simulink model "MSM_strain_wave_actuator"  (R2024b)
settings: Solver=ode23t  StartTime=0.0  StopTime=SIMULATION_TIME  FixedStep=MAX_TIME_STEP  MaxStep=MAX_TIME_STEP  RelTol=1e-3  AbsTol=1e-3  EnableMultiTasking=on
PreLoadFcn:
  | linear_mechanism = Simulink.Variant('motion_type == "linear"');
  | rotary_mechanism = Simulink.Variant('motion_type == "rotary"');
values from neighbouring files (symbols this model uses):
  action = round(out.position_data.Data(:,5))    [msm_tooth_training_run.m]
  contact_ratio = tooth_plates_cnt / (2 * (t_a / t_b + 1))    (= 2)    [MSM_mechanism_simulation_properties.m]
  contraction_initial = -msm_length * e_initial    (= -0.001)    [MSM_mechanism_simulation_properties.m]
  controller_type_vec = zeros(tooth_plates_cnt, 1)    [MSM_mechanism_simulation_properties.m]
  controller_velocity_setpoint = velocity_iter    [controller_mass_comparison_runs.m]
  disk_diameter = disk_teeth_count * tooth_pitch / pi    [MSM_mechanism_simulation_properties.m]    (also in msm_sim_runs_for_pid.m = evalin('base','disk_diameter'); save_sim_result.m = evalin('base','disk_diameter'))
  disk_height = 2.5e-4    (= 0.00025)    [MSM_mechanism_simulation_properties.m]    (also in get_tooth_properties.m)
  feedback_threshold = 1.025    [MSM_mechanism_simulation_properties.m]    (also in get_tooth_properties.m; msm_sim_runs_for_pid.m = evalin('base','feedback_threshold'))
  force_control_coeff = 1.0    (= 1)    [MSM_mechanism_simulation_properties.m]
  HALT_VELOCITY = 0.2    [MSM_mechanism_simulation_properties.m]    (also in get_tooth_properties.m)
  in_pair_angle_tooth_plates_pitch = 2*pi * (-2*tooth_pitch + in_pair_tooth_plates_pitch) / (pi*disk_diameter)    (= 0.412285714286)    [MSM_mechanism_simulation_properties.m]    (also in get_tooth_properties.m = 2*pi * (-2*tooth_pitch + in_pair_tooth_plates_pitch) / (pi*t)
  MAX_OVERLOAD_VELOCITY = 100    [MSM_mechanism_simulation_properties.m]    (also in get_tooth_properties.m)
  MAX_POSITION = rack_initial_position + max_teeth_passed * tooth_plates_cnt * angle_single_tooth_step    [MSM_mechanism_simulation_properties.m]    (also in get_tooth_properties.m)
  MAX_TIME_STEP = 5e-6    (= 5e-06)    [MSM_mechanism_simulation_properties.m]
  min_tooth_motion_range = -msm_length * allowed_elongation    (= -0.001)    [MSM_mechanism_simulation_properties.m]
  motion_type_number = NaN    [MSM_mechanism_simulation_properties.m]
  next_vec_fraction = -0.05    [MSM_mechanism_simulation_properties.m]    (also in msm_sim_runs_for_pid.m = evalin('base','next_vec_fraction'))
  obs_matrix = zeros(tooth_plates_cnt, obs_matrix_size)    [MSM_mechanism_simulation_properties.m]
  one_side_absolute_offset = one_side_elongation_capacity * msm_length    (= 0.0001)    [MSM_mechanism_simulation_properties.m]
  rack_coulumb_friction = 0.05    [MSM_mechanism_simulation_properties.m]
  rack_initial_position = rack_initial_position + 4*angle_single_tooth_step    (= 0.0554357142857)    [MSM_mechanism_simulation_properties.m]    (also in get_tooth_properties.m = rack_initial_position + 4*angle_single_tooth_step)
  rack_mass = 4e-3    (= 0.004)    [MSM_mechanism_simulation_properties.m]
  rotational_rack_coulumb_friction = rack_coulumb_friction * disk_diameter    (= 0.00175)    [MSM_mechanism_simulation_properties.m]
  SIMULATION_TIME = 0.06    [MSM_mechanism_simulation_properties.m]    (also in msm_actuation_time_sensetivity.m = 0.04; msm_sim_runs_for_pid.m = evalin('base','SIMULATION_TIME'); msm_simulation_run.m = 0.08; msm_tooth_training_run.m = 0.04)
  swing_block_tooth_plates_pitch = 2 * tooth_pitch * 22 + tooth_pitch / tooth_plates_cnt    (= 0.0172575)    [MSM_mechanism_simulation_properties.m]    (also in get_tooth_properties.m = 2 * tooth_pitch * 22 + tooth_pitch / tooth_plates_cnt)
  tooth_disk_mass = 5e-3    (= 0.005)    [MSM_mechanism_simulation_properties.m]
  tooth_pitch = tooth_pitch * tooth_size_modifier    (= 0.00039)    [MSM_mechanism_simulation_properties.m]    (also in get_tooth_properties.m = 0.00024661; msm_sim_runs_for_pid.m = evalin('base','tooth_pitch'); save_sim_result.m = evalin('base','tooth_pitch'))
  tooth_plates_cnt = 4    [MSM_mechanism_simulation_properties.m]    (also in MSM_simulation_data_processing.m = sim_data.tooth_plates_cnt; msm_actuation_time_sensetivity.m = plates_cnt_iter; msm_sim_runs_for_pid.m = evalin('base','tooth_plates_cnt'); msm_simulation_run.m = plates_cnt_iter)
  tooth_plates_pitch = tooth_pitch * 12 + tooth_pitch / tooth_plates_cnt    (= 0.0047775)    [MSM_mechanism_simulation_properties.m]    (also in get_tooth_properties.m = tooth_pitch * 12 + tooth_pitch / tooth_plates_cnt)
  useful_load = -2    [MSM_mechanism_simulation_properties.m]    (also in controller_mass_comparison_runs.m)
  useful_mass = 0.0001    [MSM_mechanism_simulation_properties.m]    (also in controller_mass_comparison_runs.m = 0.025)
  VALIDATION_START_TIME = 0.25*SIMULATION_TIME    (= 0.015)    [MSM_mechanism_simulation_properties.m]
  Z = griddata(x,y,z,X,Y)    [MSM_simulation_data_processing.m]
undefined symbols (not defined in the file or in its folder): controller_amplitude_setpoint, controller_desired_profile_type, controller_frequency_setpoint, controller_loop_type, enable_neighbours_obs, enable_vel_setpoint, external_control_value, has_external_controller, initial_spike_force, random_delay_probablity, random_switch_probability, sim_state_code, simulation_pause_time, X, Y
libraries: sm_lib x141, MSM_element x72, Flat_tooth_plate x36, Rotary_tooth_plate x36, Swing_mechanism x18, nesl_utility x16, simulink x10, fl_lib x9, rllib x7, spsMeanLib x2, slctrl_autotuning x2, slpidlib x1
(part 4 of 7)

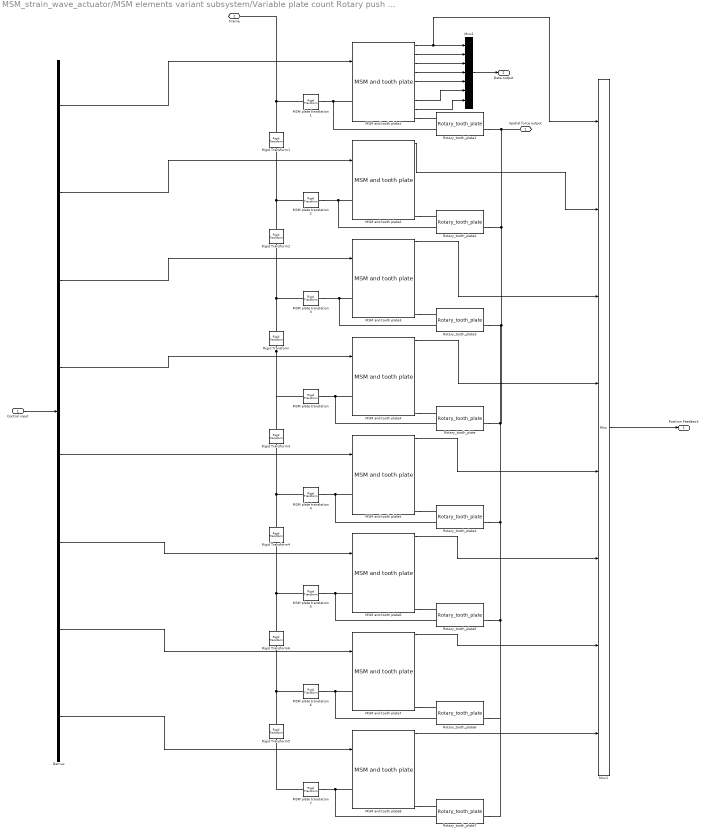
== system MSM_strain_wave_actuator/MSM elements variant subsystem/Variable plate count Rotary push spring plates/Rotary push spring 8 plates ==
  Control input : Inport
  Demux : Demux  Outputs=8
  MSM and tooth plate{1..8} (8 alike) : MSM_element/MSM and tooth plate  PositionTargetValue=contraction_initial
  MSM plate translation{,1..7} (8 alike) : sm_lib/Frames and Transforms/Rigid Transform  TranslationMethod=StandardAxis  TranslationStandardOffset=disk_diameter / 2  TranslationStandardOffsetUnits=m  TranslationStandardAxis=+Y  TranslationCartesianOffset=[0 0 0]  TranslationCartesianOffsetUnits=m  TranslationROffset=0  TranslationROffsetUnits=m  TranslationZOffset=0  TranslationZOffsetUnits=m  TranslationThetaOffset=0  TranslationThetaOffsetUnits=deg  RotationMethod=StandardAxis  RotationAngleUnits=deg  RotationStandardAxis=-X  RotationAngle=90  RotationArbitraryAxis=[0 0 1]  FollAlignAxisA=+X  BaseAlignAxisA=+Y  FollAlignAxisB=+Y  BaseAlignAxisB=+Z  RotationSequenceAxes=FollowerAxes  RotationSequence=XYX  RotationSequenceAngles=[0 0 0]  RotationSequenceAnglesUnits=deg  RotationMatrix=[1 0 0; 0 1 0; 0 0 1]  Quaternion=[1 0 0 0]
  Mux1 : Mux  Inputs=8
  Mux2 : Mux  Inputs=7
  Rigid Transform{,1..6} (7 alike) : sm_lib/Frames and Transforms/Rigid Transform  TranslationMethod=None  TranslationStandardOffset=0  TranslationStandardOffsetUnits=m  TranslationStandardAxis=+Z  TranslationCartesianOffset=[0 0 0]  TranslationCartesianOffsetUnits=m  TranslationROffset=0  TranslationROffsetUnits=m  TranslationZOffset=0  TranslationZOffsetUnits=m  TranslationThetaOffset=0  TranslationThetaOffsetUnits=deg  RotationMethod=StandardAxis  RotationAngleUnits=rad  RotationStandardAxis=+Z  RotationAngle=angle_tooth_plates_pitch  RotationArbitraryAxis=[0 0 1]  FollAlignAxisA=+X  BaseAlignAxisA=+Y  FollAlignAxisB=+Y  BaseAlignAxisB=+Z  RotationSequenceAxes=FollowerAxes  RotationSequence=XYX  RotationSequenceAngles=[0 0 0]  RotationSequenceAnglesUnits=deg  RotationMatrix=[1 0 0; 0 1 0; 0 0 1]  Quaternion=[1 0 0 0]
  Rotary_tooth_plate{,1..7} (8 alike) : Rotary_tooth_plate/Rotary_tooth_plate  SystemSampleTime=-1  VariantActivationTime=update diagram  AllowFlexibleInterface=on  Latency=0  AutoFrameSizeCalculation=off
  Spatial force output : PMIOPort  Side=Right
  Frame : PMIOPort  Port=2  Side=Left
  Position Feedback : Outport
  Data output : Outport  Port=2
  wires:
  Demux/4 -> MSM and tooth plate4/1
  MSM and tooth plate2/1 -> Mux1/2
  Control input/1 -> Demux/1
  Mux1/1 -> Position Feedback/1
  Demux/3 -> MSM and tooth plate3/1
  MSM and tooth plate4/1 -> Mux1/4
  Demux/1 -> MSM and tooth plate1/1
  Demux/2 -> MSM and tooth plate2/1
  MSM and tooth plate3/1 -> Mux1/3
  MSM and tooth plate1/1 -> Mux2/1, Mux1/1
  Demux/5 -> MSM and tooth plate5/1
  Demux/6 -> MSM and tooth plate6/1
  MSM and tooth plate5/1 -> Mux1/5
  MSM and tooth plate6/1 -> Mux1/6
  Demux/7 -> MSM and tooth plate7/1
  Demux/8 -> MSM and tooth plate8/1
  MSM and tooth plate7/1 -> Mux1/7
  MSM and tooth plate8/1 -> Mux1/8
  Mux2/1 -> Data output/1
  MSM and tooth plate1/2 -> Mux2/2
  MSM and tooth plate1/3 -> Mux2/3
  MSM and tooth plate1/4 -> Mux2/4
  MSM and tooth plate1/5 -> Mux2/5
  MSM and tooth plate1/7 -> Mux2/6
  MSM and tooth plate1/8 -> Mux2/7
  connections:
  MSM plate translation/RConn1 -- Rotary_tooth_plate/LConn2 -- MSM and tooth plate4/LConn1
  MSM plate translation3/LConn1 -- Rigid Transform/LConn1 -- Rigid Transform2/RConn1
  MSM plate translation1/LConn1 -- Frame/RConn1 -- Rigid Transform1/LConn1
  Rotary_tooth_plate1/RConn1 -- Spatial force output/RConn1 -- Rotary_tooth_plate2/RConn1 -- Rotary_tooth_plate3/RConn1 -- Rotary_tooth_plate/RConn1 -- Rotary_tooth_plate7/RConn1 -- Rotary_tooth_plate6/RConn1 -- Rotary_tooth_plate5/RConn1 -- Rotary_tooth_plate4/RConn1
  MSM and tooth plate4/RConn1 -- Rotary_tooth_plate/LConn1
  MSM and tooth plate1/RConn1 -- Rotary_tooth_plate1/LConn1
  Rotary_tooth_plate1/LConn2 -- MSM plate translation1/RConn1 -- MSM and tooth plate1/LConn1
  MSM plate translation2/LConn1 -- Rigid Transform2/LConn1 -- Rigid Transform1/RConn1
  MSM and tooth plate2/RConn1 -- Rotary_tooth_plate2/LConn1
  Rigid Transform/RConn1 -- MSM plate translation/LConn1 -- Rigid Transform3/LConn1
  MSM and tooth plate3/RConn1 -- Rotary_tooth_plate3/LConn1
  MSM plate translation3/RConn1 -- Rotary_tooth_plate3/LConn2 -- MSM and tooth plate3/LConn1
  MSM plate translation2/RConn1 -- Rotary_tooth_plate2/LConn2 -- MSM and tooth plate2/LConn1
  Rotary_tooth_plate4/LConn2 -- MSM and tooth plate5/LConn1 -- MSM plate translation4/RConn1
  Rigid Transform4/LConn1 -- MSM plate translation4/LConn1 -- Rigid Transform3/RConn1
  MSM and tooth plate5/RConn1 -- Rotary_tooth_plate4/LConn1
  Rotary_tooth_plate5/LConn2 -- MSM and tooth plate6/LConn1 -- MSM plate translation5/RConn1
  MSM plate translation5/LConn1 -- Rigid Transform6/LConn1 -- Rigid Transform4/RConn1
  MSM and tooth plate6/RConn1 -- Rotary_tooth_plate5/LConn1
  MSM plate translation6/LConn1 -- Rigid Transform5/LConn1 -- Rigid Transform6/RConn1
  MSM plate translation7/RConn1 -- Rotary_tooth_plate7/LConn2 -- MSM and tooth plate8/LConn1
  MSM plate translation6/RConn1 -- Rotary_tooth_plate6/LConn2 -- MSM and tooth plate7/LConn1
  MSM plate translation7/LConn1 -- Rigid Transform5/RConn1
  MSM and tooth plate8/RConn1 -- Rotary_tooth_plate7/LConn1
  MSM and tooth plate7/RConn1 -- Rotary_tooth_plate6/LConn1

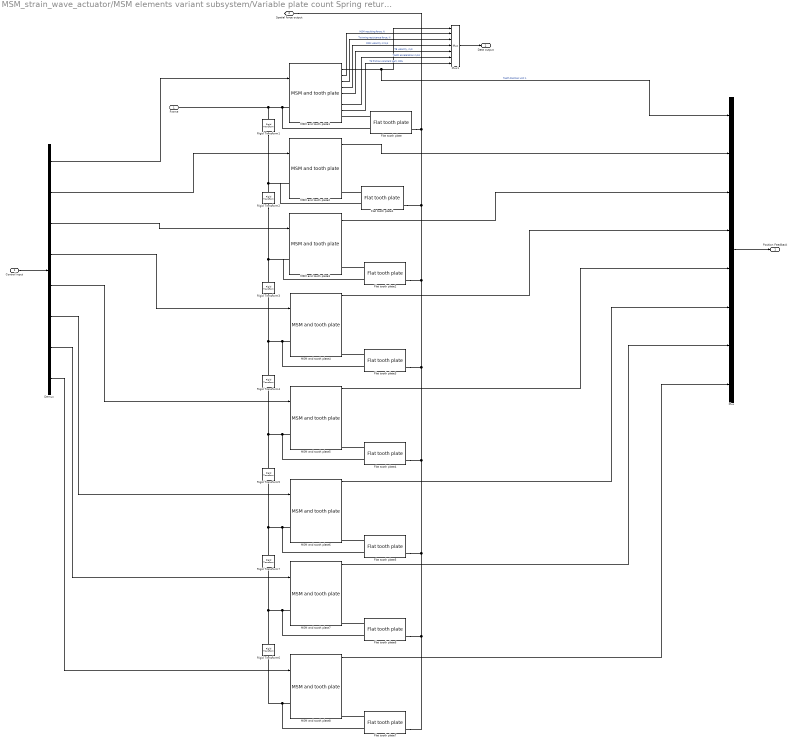
== system MSM_strain_wave_actuator/MSM elements variant subsystem/Variable plate count Spring returned plates/eight_tooth_plates ==
  Control input : Inport
  Demux : Demux  Outputs=8
  Flat tooth plate{,1..7} (8 alike) : Flat_tooth_plate/Flat tooth plate  SystemSampleTime=-1  VariantActivationTime=update diagram  AllowFlexibleInterface=on  Latency=0  AutoFrameSizeCalculation=off
  MSM and tooth plate1 : MSM_element/MSM and tooth plate  PositionTargetValue=contraction_initial * 0.15
  MSM and tooth plate2 : MSM_element/MSM and tooth plate  PositionTargetValue=contraction_initial * 0.5
  MSM and tooth plate3 : MSM_element/MSM and tooth plate  PositionTargetValue=contraction_initial * 0.9
  MSM and tooth plate{4..8} (5 alike) : MSM_element/MSM and tooth plate  PositionTargetValue=contraction_initial
  Mux : Mux  Inputs=8
  Mux1 : Mux  Inputs=7
  Rigid Transform{1..7} (7 alike) : sm_lib/Frames and Transforms/Rigid Transform  RotationMethod=None  FollAlignAxisA=+X  BaseAlignAxisA=+Y  FollAlignAxisB=+Y  BaseAlignAxisB=+Z  RotationStandardAxis=+Z  RotationAngle=0.0  RotationAngleUnits=deg  RotationArbitraryAxis=[0 0 1]  RotationSequenceAxes=FollowerAxes  RotationSequence=XYX  RotationSequenceAngles=[0 0 0]  RotationSequenceAnglesUnits=deg  RotationMatrix=[1 0 0; 0 1 0; 0 0 1]  Quaternion=[1 0 0 0]  TranslationMethod=Cartesian  TranslationCartesianOffset=[tooth_plates_pitch 0 0]  TranslationCartesianOffsetUnits=m  TranslationStandardAxis=+Z  TranslationStandardOffset=0  TranslationStandardOffsetUnits=m  TranslationROffset=0  TranslationROffsetUnits=m  TranslationThetaOffset=0  TranslationThetaOffsetUnits=deg  TranslationZOffset=0  TranslationZOffsetUnits=m
  Frame : PMIOPort  Side=Left
  Spatial force output : PMIOPort  Port=2  Side=Right
  Position Feedback : Outport
  Data output : Outport  Port=2
  wires:
  Control input/1 -> Demux/1
  Demux/4 -> MSM and tooth plate4/1
  Demux/3 -> MSM and tooth plate3/1
  MSM and tooth plate2/1 -> Mux/2
  Demux/1 -> MSM and tooth plate1/1
  Demux/2 -> MSM and tooth plate2/1
  MSM and tooth plate4/1 -> Mux/4
  MSM and tooth plate1/1 -> Mux1/1, Mux/1  "Tooth Position Unit 1"
  MSM and tooth plate3/1 -> Mux/3
  Mux/1 -> Position Feedback/1
  Demux/5 -> MSM and tooth plate5/1
  MSM and tooth plate5/1 -> Mux/5
  Demux/6 -> MSM and tooth plate6/1
  MSM and tooth plate6/1 -> Mux/6
  MSM and tooth plate1/2 -> Mux1/2  "MSM resulting force, N"
  MSM and tooth plate1/3 -> Mux1/3  "Twinning resistance force, N"
  MSM and tooth plate1/4 -> Mux1/4  "MSM velocity mm/s"
  MSM and tooth plate1/5 -> Mux1/5  "TB velocity, m/s"
  MSM and tooth plate1/7 -> Mux1/6  "Tooth acceleration m/ss"
  MSM and tooth plate1/8 -> Mux1/7  "TS friction constant part, MPa"
  Mux1/1 -> Data output/1
  Demux/8 -> MSM and tooth plate8/1
  Demux/7 -> MSM and tooth plate7/1
  MSM and tooth plate7/1 -> Mux/7
  MSM and tooth plate8/1 -> Mux/8
  connections:
  Flat tooth plate1/LConn1 -- MSM and tooth plate2/RConn1
  Rigid Transform2/RConn1 -- Rigid Transform3/LConn1 -- MSM and tooth plate3/LConn1 -- Flat tooth plate2/LConn2
  Rigid Transform1/RConn1 -- Rigid Transform2/LConn1 -- MSM and tooth plate2/LConn1 -- Flat tooth plate1/LConn2
  MSM and tooth plate4/LConn1 -- Flat tooth plate3/LConn2 -- Rigid Transform4/LConn1 -- Rigid Transform3/RConn1
  Flat tooth plate7/RConn1 -- Flat tooth plate/RConn1 -- Spatial force output/RConn1 -- Flat tooth plate1/RConn1 -- Flat tooth plate2/RConn1 -- Flat tooth plate3/RConn1 -- Flat tooth plate4/RConn1 -- Flat tooth plate5/RConn1 -- Flat tooth plate6/RConn1
  Flat tooth plate/LConn2 -- MSM and tooth plate1/LConn1 -- Rigid Transform1/LConn1 -- Frame/RConn1
  Flat tooth plate/LConn1 -- MSM and tooth plate1/RConn1
  Flat tooth plate2/LConn1 -- MSM and tooth plate3/RConn1
  Flat tooth plate3/LConn1 -- MSM and tooth plate4/RConn1
  Flat tooth plate4/LConn2 -- Rigid Transform5/LConn1 -- Rigid Transform4/RConn1 -- MSM and tooth plate5/LConn1
  Flat tooth plate4/LConn1 -- MSM and tooth plate5/RConn1
  Flat tooth plate5/LConn2 -- MSM and tooth plate6/LConn1 -- Rigid Transform7/LConn1 -- Rigid Transform5/RConn1
  Flat tooth plate5/LConn1 -- MSM and tooth plate6/RConn1
  MSM and tooth plate8/LConn1 -- Flat tooth plate7/LConn2 -- Rigid Transform6/RConn1
  Flat tooth plate6/LConn1 -- MSM and tooth plate7/RConn1
  Flat tooth plate7/LConn1 -- MSM and tooth plate8/RConn1
  Flat tooth plate6/LConn2 -- Rigid Transform6/LConn1 -- Rigid Transform7/RConn1 -- MSM and tooth plate7/LConn1

== system MSM_strain_wave_actuator/MSM elements variant subsystem/Variable plate count Spring returned plates/four_tooth_plates ==
  Control input : Inport
  Demux : Demux
  Flat tooth plate{,1..3} (4 alike) : Flat_tooth_plate/Flat tooth plate  SystemSampleTime=-1  VariantActivationTime=update diagram  AllowFlexibleInterface=on  Latency=0  AutoFrameSizeCalculation=off
  MSM and tooth plate1 : MSM_element/MSM and tooth plate  PositionTargetValue=contraction_initial * 0.8
  MSM and tooth plate2 : MSM_element/MSM and tooth plate  PositionTargetValue=contraction_initial * 0.8
  MSM and tooth plate3 : MSM_element/MSM and tooth plate  PositionTargetValue=contraction_initial
  MSM and tooth plate4 : MSM_element/MSM and tooth plate  PositionTargetValue=contraction_initial
  Mux : Mux
  Mux1 : Mux  Inputs=7
  Rigid Transform1 : sm_lib/Frames and Transforms/Rigid Transform  RotationMethod=None  FollAlignAxisA=+X  BaseAlignAxisA=+Y  FollAlignAxisB=+Y  BaseAlignAxisB=+Z  RotationStandardAxis=+Z  RotationAngle=0.0  RotationAngleUnits=deg  RotationArbitraryAxis=[0 0 1]  RotationSequenceAxes=FollowerAxes  RotationSequence=XYX  RotationSequenceAngles=[0 0 0]  RotationSequenceAnglesUnits=deg  RotationMatrix=[1 0 0; 0 1 0; 0 0 1]  Quaternion=[1 0 0 0]  TranslationMethod=Cartesian  TranslationCartesianOffset=[tooth_plates_pitch 0 0]  TranslationCartesianOffsetUnits=m  TranslationStandardAxis=+Z  TranslationStandardOffset=0  TranslationStandardOffsetUnits=m  TranslationROffset=0  TranslationROffsetUnits=m  TranslationThetaOffset=0  TranslationThetaOffsetUnits=deg  TranslationZOffset=0  TranslationZOffsetUnits=m
  Rigid Transform2 : sm_lib/Frames and Transforms/Rigid Transform  RotationMethod=None  FollAlignAxisA=+X  BaseAlignAxisA=+Y  FollAlignAxisB=+Y  BaseAlignAxisB=+Z  RotationStandardAxis=+Z  RotationAngle=0.0  RotationAngleUnits=deg  RotationArbitraryAxis=[0 0 1]  RotationSequenceAxes=FollowerAxes  RotationSequence=XYX  RotationSequenceAngles=[0 0 0]  RotationSequenceAnglesUnits=deg  RotationMatrix=[1 0 0; 0 1 0; 0 0 1]  Quaternion=[1 0 0 0]  TranslationMethod=Cartesian  TranslationCartesianOffset=[tooth_plates_pitch 0 0]  TranslationCartesianOffsetUnits=m  TranslationStandardAxis=+Z  TranslationStandardOffset=0  TranslationStandardOffsetUnits=m  TranslationROffset=0  TranslationROffsetUnits=m  TranslationThetaOffset=0  TranslationThetaOffsetUnits=deg  TranslationZOffset=0  TranslationZOffsetUnits=m
  Rigid Transform3 : sm_lib/Frames and Transforms/Rigid Transform  RotationMethod=None  FollAlignAxisA=+X  BaseAlignAxisA=+Y  FollAlignAxisB=+Y  BaseAlignAxisB=+Z  RotationStandardAxis=+Z  RotationAngle=0.0  RotationAngleUnits=deg  RotationArbitraryAxis=[0 0 1]  RotationSequenceAxes=FollowerAxes  RotationSequence=XYX  RotationSequenceAngles=[0 0 0]  RotationSequenceAnglesUnits=deg  RotationMatrix=[1 0 0; 0 1 0; 0 0 1]  Quaternion=[1 0 0 0]  TranslationMethod=Cartesian  TranslationCartesianOffset=[tooth_plates_pitch 0 0]  TranslationCartesianOffsetUnits=m  TranslationStandardAxis=+Z  TranslationStandardOffset=0  TranslationStandardOffsetUnits=m  TranslationROffset=0  TranslationROffsetUnits=m  TranslationThetaOffset=0  TranslationThetaOffsetUnits=deg  TranslationZOffset=0  TranslationZOffsetUnits=m
  Frame : PMIOPort  Side=Left
  Spatial force output : PMIOPort  Port=2  Side=Right
  Position Feedback : Outport
  Data output : Outport  Port=2
  wires:
  Control input/1 -> Demux/1
  Demux/4 -> MSM and tooth plate4/1
  Demux/3 -> MSM and tooth plate3/1
  MSM and tooth plate2/1 -> Mux/2
  Demux/1 -> MSM and tooth plate1/1
  Demux/2 -> MSM and tooth plate2/1
  MSM and tooth plate4/1 -> Mux/4
  MSM and tooth plate1/1 -> Mux1/1, Mux/1  "Tooth Position Unit 1"
  MSM and tooth plate3/1 -> Mux/3
  Mux/1 -> Position Feedback/1
  MSM and tooth plate1/2 -> Mux1/2  "MSM resulting force, N"
  MSM and tooth plate1/3 -> Mux1/3  "Twinning resistance force, N"
  MSM and tooth plate1/4 -> Mux1/4  "MSM velocity mm/s"
  MSM and tooth plate1/5 -> Mux1/5  "TB velocity, m/s"
  MSM and tooth plate1/7 -> Mux1/6  "Tooth acceleration m/ss"
  MSM and tooth plate1/8 -> Mux1/7  "TS friction constant part, MPa"
  Mux1/1 -> Data output/1
  connections:
  Flat tooth plate1/LConn1 -- MSM and tooth plate2/RConn1
  Rigid Transform2/RConn1 -- Rigid Transform3/LConn1 -- MSM and tooth plate3/LConn1 -- Flat tooth plate2/LConn2
  Rigid Transform1/RConn1 -- Rigid Transform2/LConn1 -- MSM and tooth plate2/LConn1 -- Flat tooth plate1/LConn2
  MSM and tooth plate4/LConn1 -- Flat tooth plate3/LConn2 -- Rigid Transform3/RConn1
  Flat tooth plate/RConn1 -- Flat tooth plate3/RConn1 -- Flat tooth plate2/RConn1 -- Flat tooth plate1/RConn1 -- Spatial force output/RConn1
  Flat tooth plate/LConn2 -- MSM and tooth plate1/LConn1 -- Rigid Transform1/LConn1 -- Frame/RConn1
  Flat tooth plate/LConn1 -- MSM and tooth plate1/RConn1
  Flat tooth plate2/LConn1 -- MSM and tooth plate3/RConn1
  Flat tooth plate3/LConn1 -- MSM and tooth plate4/RConn1

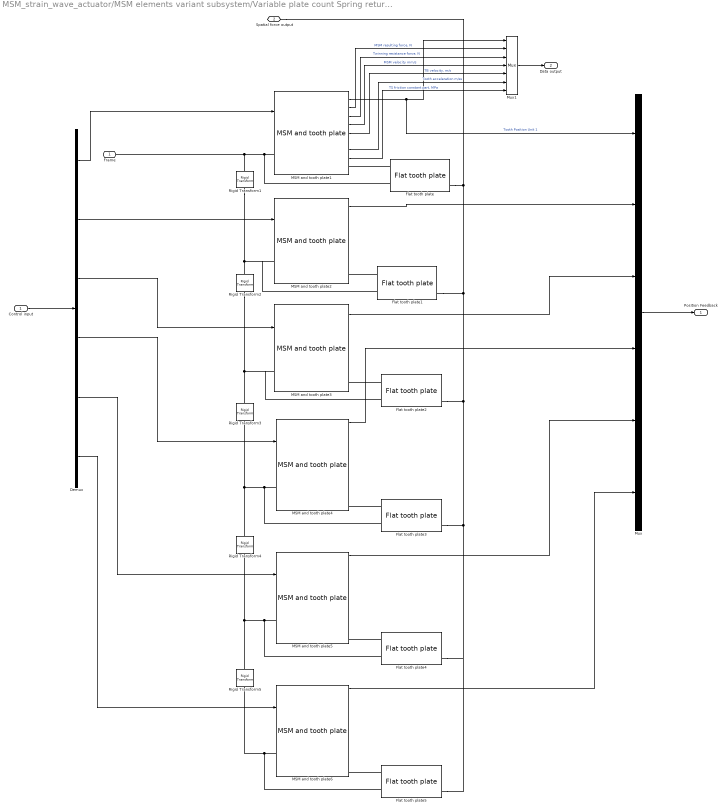
== system MSM_strain_wave_actuator/MSM elements variant subsystem/Variable plate count Spring returned plates/six_tooth_plates ==
  Control input : Inport
  Demux : Demux  Outputs=6
  Flat tooth plate{,1..5} (6 alike) : Flat_tooth_plate/Flat tooth plate  SystemSampleTime=-1  VariantActivationTime=update diagram  AllowFlexibleInterface=on  Latency=0  AutoFrameSizeCalculation=off
  MSM and tooth plate1 : MSM_element/MSM and tooth plate  PositionTargetValue=contraction_initial*0.2
  MSM and tooth plate2 : MSM_element/MSM and tooth plate  PositionTargetValue=contraction_initial*0.55
  MSM and tooth plate{3..6} (4 alike) : MSM_element/MSM and tooth plate  PositionTargetValue=contraction_initial
  Mux : Mux  Inputs=6
  Mux1 : Mux  Inputs=7
  Rigid Transform{1..5} (5 alike) : sm_lib/Frames and Transforms/Rigid Transform  TranslationMethod=Cartesian  TranslationStandardOffset=0  TranslationStandardOffsetUnits=m  TranslationStandardAxis=+Z  TranslationCartesianOffset=[tooth_plates_pitch 0 0]  TranslationCartesianOffsetUnits=m  TranslationROffset=0  TranslationROffsetUnits=m  TranslationZOffset=0  TranslationZOffsetUnits=m  TranslationThetaOffset=0  TranslationThetaOffsetUnits=deg  RotationMethod=None  RotationAngleUnits=deg  RotationStandardAxis=+Z  RotationAngle=0.0  RotationArbitraryAxis=[0 0 1]  FollAlignAxisA=+X  BaseAlignAxisA=+Y  FollAlignAxisB=+Y  BaseAlignAxisB=+Z  RotationSequenceAxes=FollowerAxes  RotationSequence=XYX  RotationSequenceAngles=[0 0 0]  RotationSequenceAnglesUnits=deg  RotationMatrix=[1 0 0; 0 1 0; 0 0 1]  Quaternion=[1 0 0 0]
  Frame : PMIOPort  Side=Left
  Spatial force output : PMIOPort  Port=2  Side=Right
  Position Feedback : Outport
  Data output : Outport  Port=2
  wires:
  Control input/1 -> Demux/1
  Demux/4 -> MSM and tooth plate4/1
  Demux/3 -> MSM and tooth plate3/1
  MSM and tooth plate2/1 -> Mux/2
  Demux/1 -> MSM and tooth plate1/1
  Demux/2 -> MSM and tooth plate2/1
  MSM and tooth plate4/1 -> Mux/4
  MSM and tooth plate1/1 -> Mux1/1, Mux/1  "Tooth Position Unit 1"
  MSM and tooth plate3/1 -> Mux/3
  Mux/1 -> Position Feedback/1
  Demux/5 -> MSM and tooth plate5/1
  MSM and tooth plate5/1 -> Mux/5
  Demux/6 -> MSM and tooth plate6/1
  MSM and tooth plate6/1 -> Mux/6
  MSM and tooth plate1/2 -> Mux1/2  "MSM resulting force, N"
  MSM and tooth plate1/3 -> Mux1/3  "Twinning resistance force, N"
  MSM and tooth plate1/4 -> Mux1/4  "MSM velocity mm/s"
  MSM and tooth plate1/5 -> Mux1/5  "TB velocity, m/s"
  MSM and tooth plate1/7 -> Mux1/6  "Tooth acceleration m/ss"
  MSM and tooth plate1/8 -> Mux1/7  "TS friction constant part, MPa"
  Mux1/1 -> Data output/1
  connections:
  Flat tooth plate1/LConn1 -- MSM and tooth plate2/RConn1
  Rigid Transform2/RConn1 -- Rigid Transform3/LConn1 -- MSM and tooth plate3/LConn1 -- Flat tooth plate2/LConn2
  Rigid Transform1/RConn1 -- Rigid Transform2/LConn1 -- MSM and tooth plate2/LConn1 -- Flat tooth plate1/LConn2
  MSM and tooth plate4/LConn1 -- Flat tooth plate3/LConn2 -- Rigid Transform4/LConn1 -- Rigid Transform3/RConn1
  Flat tooth plate/RConn1 -- Flat tooth plate4/RConn1 -- Flat tooth plate5/RConn1 -- Flat tooth plate3/RConn1 -- Flat tooth plate2/RConn1 -- Flat tooth plate1/RConn1 -- Spatial force output/RConn1
  Flat tooth plate/LConn2 -- MSM and tooth plate1/LConn1 -- Rigid Transform1/LConn1 -- Frame/RConn1
  Flat tooth plate/LConn1 -- MSM and tooth plate1/RConn1
  Flat tooth plate2/LConn1 -- MSM and tooth plate3/RConn1
  Flat tooth plate3/LConn1 -- MSM and tooth plate4/RConn1
  Flat tooth plate4/LConn2 -- Rigid Transform5/LConn1 -- Rigid Transform4/RConn1 -- MSM and tooth plate5/LConn1
  Flat tooth plate4/LConn1 -- MSM and tooth plate5/RConn1
  Flat tooth plate5/LConn2 -- Rigid Transform5/RConn1 -- MSM and tooth plate6/LConn1
  Flat tooth plate5/LConn1 -- MSM and tooth plate6/RConn1

== system MSM_strain_wave_actuator/controller/Check if actuator halted or overloaded or reached max position/Save scalar result ==
  stop_sim_code : Inport
  Enable : EnablePort
  To Workspace : ToWorkspace  VariableName=sim_stop_result  SaveFormat=Timeseries  SampleTime=-1
  wires:
  stop_sim_code/1 -> To Workspace/1

== system MSM_strain_wave_actuator/controller/Old controller/Check if actuator halted or overloaded or reached max position1 ==
  cur_rack_position : Inport
  is_load_applied : Inport  Port=2
  Abs : Abs  Commented=on  SaturateOnIntegerOverflow=off
  Check sim stop conditions : MATLAB Function  TreatAsAtomicUnit=on
  Clock1 : Clock
  Compare To Constant : simulink/Logic and Bit Operations/Compare To Constant  relop=>=  const=0.5  OutDataTypeStr=boolean
  Compare To Constant1 : simulink/Logic and Bit Operations/Compare To Constant  relop=>=  const=0.5  OutDataTypeStr=boolean
  Constant : Constant  Commented=on  Value=rack_initial_position
  DISABLED FOR NN TRAINING Stop Simulation : Stop  Commented=on
  Delay : Delay  DelayLength=1  InitialCondition=NaN
  Delay1 : Delay
  Mean : spsMeanLib/Mean  Commented=on  Freq=1 / (SIMULATION_TIME * 0.05)  Vinit=0  Ts=0
  Save scalar result : Subsystem  TreatAsAtomicUnit=on
  stop_sim_code : Outport
  wires:
  Compare To Constant1/1 -> Check sim stop conditions/1(is_load_applied)
  Clock1/1 -> Check sim stop conditions/2(time)
  is_load_applied/1 -> Compare To Constant1/1
  Abs/1 -> Mean/1
  Check sim stop conditions/1(stop_sim_code) -> Delay1/1, stop_sim_code/1
  cur_rack_position/1 -> Check sim stop conditions/3(rack_cur_pos)
  Delay/1 -> Check sim stop conditions/4(memory_pos)
  Check sim stop conditions/3(out_pos) -> Delay/1
  Compare To Constant/1 -> DISABLED FOR NN TRAINING Stop Simulation/1, Save scalar result/Enable
  Delay1/1 -> Save scalar result/1(stop_sim_code), Compare To Constant/1

== system MSM_strain_wave_actuator/controller/Old controller/Closed//open loop simple feedback controller1 ==
  position mapping : Inport
  rack position : Inport  Port=2
  initial spike : Inport  Port=3
  Velocity setpoint : Inport  Port=4
  Clock : Clock
  Constant : Constant  Value=tooth_pitch
  Constant1 : Constant  Value=1.5*MAX_TIME_STEP
  Delay1 : Delay  DelayLength=1  InitialCondition=1
  Gain1 : Gain  Gain=force_control_coeff
  Loop type control : Constant  Value=controller_loop_type
  MATLAB Function : MATLAB Function  TreatAsAtomicUnit=on
  Velocity to frequency : Product  Inputs=*/
  Control Input : Outport
  wires:
  Constant1/1 -> MATLAB Function/4(initial_idle_time)
  Velocity to frequency/1 -> MATLAB Function/3(cycle_length)
  Loop type control/1 -> MATLAB Function/2(loop_type)
  MATLAB Function/1(output_vector) -> Gain1/1
  rack position/1 -> MATLAB Function/6(rack_position)
  MATLAB Function/2(cur_active_output) -> Delay1/1
  Delay1/1 -> MATLAB Function/8(currently_active)
  Clock/1 -> MATLAB Function/1(time)
  initial spike/1 -> MATLAB Function/7(ticks_cnt)
  position mapping/1 -> MATLAB Function/5(feedback)
  Gain1/1 -> Control Input/1
  Constant/1 -> Velocity to frequency/1
  Velocity setpoint/1 -> Velocity to frequency/2

== system MSM_strain_wave_actuator/MSM elements variant subsystem/Variable plate count Linear push push plates/Linear_swing_eight_tooth_plates/Subsystem ==
  Control input [0; 1] : Inport
  Control input [0; 1]1 : Inport  Port=2
  Flat tooth plate : Flat_tooth_plate/Flat tooth plate  SystemSampleTime=-1  VariantActivationTime=update diagram  AllowFlexibleInterface=on  Latency=0  AutoFrameSizeCalculation=off
  Flat tooth plate2 : Flat_tooth_plate/Flat tooth plate  SystemSampleTime=-1  VariantActivationTime=update diagram  AllowFlexibleInterface=on  Latency=0  AutoFrameSizeCalculation=off
  MSM and tooth plate1 : MSM_element/MSM and tooth plate  PositionTargetValue=contraction_initial * 0.4
  MSM and tooth plate3 : MSM_element/MSM and tooth plate  PositionTargetValue=contraction_initial * 0.6
  Mux1 : Mux  Inputs=7
  Swing mechanism : Swing_mechanism/Swing mechanism  SystemSampleTime=-1  VariantActivationTime=update diagram  AllowFlexibleInterface=on  Latency=0  AutoFrameSizeCalculation=off
  Conn1 : PMIOPort  Side=Left
  Spatial force output1 : PMIOPort  Port=2  Side=Right
  Tooth Position Unit 1 : Outport
  "Tooth position COUNTERPHASE, mm" : Outport  Port=2
  Data output : Outport  Port=3
  wires:
  MSM and tooth plate1/2 -> Mux1/2  "MSM resulting force, N"
  MSM and tooth plate1/8 -> Mux1/7  "TS friction constant part, MPa"
  MSM and tooth plate1/7 -> Mux1/6  "Tooth acceleration m/ss"
  MSM and tooth plate1/1 -> Tooth Position Unit 1/1, Mux1/1  "Tooth Position Unit 1"
  MSM and tooth plate1/5 -> Mux1/5  "TB velocity, m/s"
  MSM and tooth plate1/3 -> Mux1/3  "Twinning resistance force, N"
  MSM and tooth plate1/4 -> Mux1/4  "MSM velocity mm/s"
  Mux1/1 -> Data output/1
  Control input [0; 1]1/1 -> MSM and tooth plate3/1
  MSM and tooth plate3/1 -> "Tooth position COUNTERPHASE, mm"/1
  Control input [0; 1]/1 -> MSM and tooth plate1/1
  connections:
  Flat tooth plate2/LConn2 -- Swing mechanism/LConn2 -- MSM and tooth plate3/LConn1
  Flat tooth plate/LConn1 -- Swing mechanism/RConn1 -- MSM and tooth plate1/RConn1
  Flat tooth plate2/LConn1 -- Swing mechanism/RConn2 -- MSM and tooth plate3/RConn1
  Spatial force output1/RConn1 -- Flat tooth plate2/RConn1 -- Flat tooth plate/RConn1
  Flat tooth plate/LConn2 -- MSM and tooth plate1/LConn1 -- Swing mechanism/LConn1 -- Conn1/RConn1

== system MSM_strain_wave_actuator/MSM elements variant subsystem/Variable plate count Linear push push plates/Linear_swing_eight_tooth_plates/Subsystem1 ==
  Control input [0; 1] : Inport
  Control input [0; 1]1 : Inport  Port=2
  Flat tooth plate : Flat_tooth_plate/Flat tooth plate  SystemSampleTime=-1  VariantActivationTime=update diagram  AllowFlexibleInterface=on  Latency=0  AutoFrameSizeCalculation=off
  Flat tooth plate2 : Flat_tooth_plate/Flat tooth plate  SystemSampleTime=-1  VariantActivationTime=update diagram  AllowFlexibleInterface=on  Latency=0  AutoFrameSizeCalculation=off
  MSM and tooth plate1 : MSM_element/MSM and tooth plate  PositionTargetValue=contraction_initial
  MSM and tooth plate3 : MSM_element/MSM and tooth plate  PositionTargetValue=contraction_initial
  Swing mechanism : Swing_mechanism/Swing mechanism  SystemSampleTime=-1  VariantActivationTime=update diagram  AllowFlexibleInterface=on  Latency=0  AutoFrameSizeCalculation=off
  Static frame 1 : PMIOPort  Side=Left
  Spatial force output1 : PMIOPort  Port=2  Side=Right
  Tooth Position Unit 1 : Outport
  "Tooth position COUNTERPHASE, mm" : Outport  Port=2
  wires:
  MSM and tooth plate1/1 -> Tooth Position Unit 1/1  "Tooth Position Unit 1"
  Control input [0; 1]1/1 -> MSM and tooth plate3/1
  MSM and tooth plate3/1 -> "Tooth position COUNTERPHASE, mm"/1
  Control input [0; 1]/1 -> MSM and tooth plate1/1
  connections:
  MSM and tooth plate1/LConn1 -- Static frame 1/RConn1 -- Flat tooth plate/LConn2 -- Swing mechanism/LConn1
  Flat tooth plate2/LConn2 -- MSM and tooth plate3/LConn1 -- Swing mechanism/LConn2
  MSM and tooth plate1/RConn1 -- Flat tooth plate/LConn1 -- Swing mechanism/RConn1
  Flat tooth plate2/LConn1 -- MSM and tooth plate3/RConn1 -- Swing mechanism/RConn2
  Spatial force output1/RConn1 -- Flat tooth plate2/RConn1 -- Flat tooth plate/RConn1

== system MSM_strain_wave_actuator/MSM elements variant subsystem/Variable plate count Linear push push plates/Linear_swing_eight_tooth_plates/Subsystem2 ==
  Control input [0; 1] : Inport
  Control input [0; 1]1 : Inport  Port=2
  Flat tooth plate : Flat_tooth_plate/Flat tooth plate  SystemSampleTime=-1  VariantActivationTime=update diagram  AllowFlexibleInterface=on  Latency=0  AutoFrameSizeCalculation=off
  Flat tooth plate2 : Flat_tooth_plate/Flat tooth plate  SystemSampleTime=-1  VariantActivationTime=update diagram  AllowFlexibleInterface=on  Latency=0  AutoFrameSizeCalculation=off
  MSM and tooth plate1 : MSM_element/MSM and tooth plate  PositionTargetValue=contraction_initial
  MSM and tooth plate3 : MSM_element/MSM and tooth plate  PositionTargetValue=contraction_initial
  Swing mechanism : Swing_mechanism/Swing mechanism  SystemSampleTime=-1  VariantActivationTime=update diagram  AllowFlexibleInterface=on  Latency=0  AutoFrameSizeCalculation=off
  Static frame 1 : PMIOPort  Side=Left
  Spatial force output1 : PMIOPort  Port=2  Side=Right
  Tooth Position Unit 1 : Outport
  "Tooth position COUNTERPHASE, mm" : Outport  Port=2
  wires:
  MSM and tooth plate1/1 -> Tooth Position Unit 1/1  "Tooth Position Unit 1"
  Control input [0; 1]1/1 -> MSM and tooth plate3/1
  MSM and tooth plate3/1 -> "Tooth position COUNTERPHASE, mm"/1
  Control input [0; 1]/1 -> MSM and tooth plate1/1
  connections:
  MSM and tooth plate1/LConn1 -- Static frame 1/RConn1 -- Flat tooth plate/LConn2 -- Swing mechanism/LConn1
  Flat tooth plate2/LConn2 -- MSM and tooth plate3/LConn1 -- Swing mechanism/LConn2
  MSM and tooth plate1/RConn1 -- Flat tooth plate/LConn1 -- Swing mechanism/RConn1
  Flat tooth plate2/LConn1 -- MSM and tooth plate3/RConn1 -- Swing mechanism/RConn2
  Spatial force output1/RConn1 -- Flat tooth plate2/RConn1 -- Flat tooth plate/RConn1

== system MSM_strain_wave_actuator/MSM elements variant subsystem/Variable plate count Linear push push plates/Linear_swing_eight_tooth_plates/Subsystem3 ==
  Control input [0; 1] : Inport
  Control input [0; 1]1 : Inport  Port=2
  Flat tooth plate : Flat_tooth_plate/Flat tooth plate  SystemSampleTime=-1  VariantActivationTime=update diagram  AllowFlexibleInterface=on  Latency=0  AutoFrameSizeCalculation=off
  Flat tooth plate2 : Flat_tooth_plate/Flat tooth plate  SystemSampleTime=-1  VariantActivationTime=update diagram  AllowFlexibleInterface=on  Latency=0  AutoFrameSizeCalculation=off
  MSM and tooth plate1 : MSM_element/MSM and tooth plate  PositionTargetValue=contraction_initial
  MSM and tooth plate3 : MSM_element/MSM and tooth plate  PositionTargetValue=contraction_initial
  Swing mechanism : Swing_mechanism/Swing mechanism  SystemSampleTime=-1  VariantActivationTime=update diagram  AllowFlexibleInterface=on  Latency=0  AutoFrameSizeCalculation=off
  Static frame 1 : PMIOPort  Side=Left
  Spatial force output1 : PMIOPort  Port=2  Side=Right
  Tooth Position Unit 1 : Outport
  "Tooth position COUNTERPHASE, mm" : Outport  Port=2
  wires:
  MSM and tooth plate1/1 -> Tooth Position Unit 1/1  "Tooth Position Unit 1"
  Control input [0; 1]1/1 -> MSM and tooth plate3/1
  MSM and tooth plate3/1 -> "Tooth position COUNTERPHASE, mm"/1
  Control input [0; 1]/1 -> MSM and tooth plate1/1
  connections:
  MSM and tooth plate1/LConn1 -- Static frame 1/RConn1 -- Flat tooth plate/LConn2 -- Swing mechanism/LConn1
  Flat tooth plate2/LConn2 -- MSM and tooth plate3/LConn1 -- Swing mechanism/LConn2
  MSM and tooth plate1/RConn1 -- Flat tooth plate/LConn1 -- Swing mechanism/RConn1
  Flat tooth plate2/LConn1 -- MSM and tooth plate3/RConn1 -- Swing mechanism/RConn2
  Spatial force output1/RConn1 -- Flat tooth plate2/RConn1 -- Flat tooth plate/RConn1

== system MSM_strain_wave_actuator/MSM elements variant subsystem/Variable plate count Linear push push plates/Linear_swing_four_tooth_plates/Subsystem ==
  Control input [0; 1] : Inport
  Control input [0; 1]1 : Inport  Port=2
  Flat tooth plate : Flat_tooth_plate/Flat tooth plate  SystemSampleTime=-1  VariantActivationTime=update diagram  AllowFlexibleInterface=on  Latency=0  AutoFrameSizeCalculation=off
  Flat tooth plate2 : Flat_tooth_plate/Flat tooth plate  SystemSampleTime=-1  VariantActivationTime=update diagram  AllowFlexibleInterface=on  Latency=0  AutoFrameSizeCalculation=off
  MSM and tooth plate1 : MSM_element/MSM and tooth plate  PositionTargetValue=contraction_initial * 0.2
  MSM and tooth plate3 : MSM_element/MSM and tooth plate  PositionTargetValue=contraction_initial * 0.8
  Mux1 : Mux  Inputs=7
  Swing mechanism : Swing_mechanism/Swing mechanism  SystemSampleTime=-1  VariantActivationTime=update diagram  AllowFlexibleInterface=on  Latency=0  AutoFrameSizeCalculation=off
  Conn1 : PMIOPort  Side=Left
  Spatial force output1 : PMIOPort  Port=2  Side=Right
  Tooth Position Unit 1 : Outport
  "Tooth position COUNTERPHASE, mm" : Outport  Port=2
  Data output : Outport  Port=3
  wires:
  MSM and tooth plate1/2 -> Mux1/2  "MSM resulting force, N"
  MSM and tooth plate1/8 -> Mux1/7  "TS friction constant part, MPa"
  MSM and tooth plate1/7 -> Mux1/6  "Tooth acceleration m/ss"
  MSM and tooth plate1/1 -> Tooth Position Unit 1/1, Mux1/1  "Tooth Position Unit 1"
  MSM and tooth plate1/5 -> Mux1/5  "TB velocity, m/s"
  MSM and tooth plate1/3 -> Mux1/3  "Twinning resistance force, N"
  MSM and tooth plate1/4 -> Mux1/4  "MSM velocity mm/s"
  Mux1/1 -> Data output/1
  Control input [0; 1]1/1 -> MSM and tooth plate3/1
  MSM and tooth plate3/1 -> "Tooth position COUNTERPHASE, mm"/1
  Control input [0; 1]/1 -> MSM and tooth plate1/1
  connections:
  Flat tooth plate2/LConn2 -- Swing mechanism/LConn2 -- MSM and tooth plate3/LConn1
  Flat tooth plate/LConn1 -- Swing mechanism/RConn1 -- MSM and tooth plate1/RConn1
  Flat tooth plate2/LConn1 -- Swing mechanism/RConn2 -- MSM and tooth plate3/RConn1
  Spatial force output1/RConn1 -- Flat tooth plate2/RConn1 -- Flat tooth plate/RConn1
  Flat tooth plate/LConn2 -- MSM and tooth plate1/LConn1 -- Swing mechanism/LConn1 -- Conn1/RConn1

== system MSM_strain_wave_actuator/MSM elements variant subsystem/Variable plate count Linear push push plates/Linear_swing_four_tooth_plates/Subsystem1 ==
  Control input [0; 1] : Inport
  Control input [0; 1]1 : Inport  Port=2
  Flat tooth plate : Flat_tooth_plate/Flat tooth plate  SystemSampleTime=-1  VariantActivationTime=update diagram  AllowFlexibleInterface=on  Latency=0  AutoFrameSizeCalculation=off
  Flat tooth plate2 : Flat_tooth_plate/Flat tooth plate  SystemSampleTime=-1  VariantActivationTime=update diagram  AllowFlexibleInterface=on  Latency=0  AutoFrameSizeCalculation=off
  MSM and tooth plate1 : MSM_element/MSM and tooth plate  PositionTargetValue=contraction_initial * 0.5
  MSM and tooth plate3 : MSM_element/MSM and tooth plate  PositionTargetValue=contraction_initial * 0.5
  Swing mechanism : Swing_mechanism/Swing mechanism  SystemSampleTime=-1  VariantActivationTime=update diagram  AllowFlexibleInterface=on  Latency=0  AutoFrameSizeCalculation=off
  Static frame 1 : PMIOPort  Side=Left
  Spatial force output1 : PMIOPort  Port=2  Side=Right
  Tooth Position Unit 1 : Outport
  "Tooth position COUNTERPHASE, mm" : Outport  Port=2
  wires:
  MSM and tooth plate1/1 -> Tooth Position Unit 1/1  "Tooth Position Unit 1"
  Control input [0; 1]1/1 -> MSM and tooth plate3/1
  MSM and tooth plate3/1 -> "Tooth position COUNTERPHASE, mm"/1
  Control input [0; 1]/1 -> MSM and tooth plate1/1
  connections:
  MSM and tooth plate1/LConn1 -- Static frame 1/RConn1 -- Flat tooth plate/LConn2 -- Swing mechanism/LConn1
  Flat tooth plate2/LConn2 -- MSM and tooth plate3/LConn1 -- Swing mechanism/LConn2
  MSM and tooth plate1/RConn1 -- Flat tooth plate/LConn1 -- Swing mechanism/RConn1
  Flat tooth plate2/LConn1 -- MSM and tooth plate3/RConn1 -- Swing mechanism/RConn2
  Spatial force output1/RConn1 -- Flat tooth plate2/RConn1 -- Flat tooth plate/RConn1

== system MSM_strain_wave_actuator/MSM elements variant subsystem/Variable plate count Linear push push plates/Linear_swing_six_tooth_plates/Subsystem ==
  Control input [0; 1] : Inport
  Control input [0; 1]1 : Inport  Port=2
  Flat tooth plate : Flat_tooth_plate/Flat tooth plate  SystemSampleTime=-1  VariantActivationTime=update diagram  AllowFlexibleInterface=on  Latency=0  AutoFrameSizeCalculation=off
  Flat tooth plate2 : Flat_tooth_plate/Flat tooth plate  SystemSampleTime=-1  VariantActivationTime=update diagram  AllowFlexibleInterface=on  Latency=0  AutoFrameSizeCalculation=off
  MSM and tooth plate1 : MSM_element/MSM and tooth plate  PositionTargetValue=contraction_initial * 0.4
  MSM and tooth plate3 : MSM_element/MSM and tooth plate  PositionTargetValue=contraction_initial * 0.6
  Mux1 : Mux  Inputs=7
  Swing mechanism : Swing_mechanism/Swing mechanism  SystemSampleTime=-1  VariantActivationTime=update diagram  AllowFlexibleInterface=on  Latency=0  AutoFrameSizeCalculation=off
  Conn1 : PMIOPort  Side=Left
  Spatial force output1 : PMIOPort  Port=2  Side=Right
  Tooth Position Unit 1 : Outport
  "Tooth position COUNTERPHASE, mm" : Outport  Port=2
  Data output : Outport  Port=3
  wires:
  MSM and tooth plate1/2 -> Mux1/2  "MSM resulting force, N"
  MSM and tooth plate1/8 -> Mux1/7  "TS friction constant part, MPa"
  MSM and tooth plate1/7 -> Mux1/6  "Tooth acceleration m/ss"
  MSM and tooth plate1/1 -> Tooth Position Unit 1/1, Mux1/1  "Tooth Position Unit 1"
  MSM and tooth plate1/5 -> Mux1/5  "TB velocity, m/s"
  MSM and tooth plate1/3 -> Mux1/3  "Twinning resistance force, N"
  MSM and tooth plate1/4 -> Mux1/4  "MSM velocity mm/s"
  Mux1/1 -> Data output/1
  Control input [0; 1]1/1 -> MSM and tooth plate3/1
  MSM and tooth plate3/1 -> "Tooth position COUNTERPHASE, mm"/1
  Control input [0; 1]/1 -> MSM and tooth plate1/1
  connections:
  Flat tooth plate2/LConn2 -- Swing mechanism/LConn2 -- MSM and tooth plate3/LConn1
  Flat tooth plate/LConn1 -- Swing mechanism/RConn1 -- MSM and tooth plate1/RConn1
  Flat tooth plate2/LConn1 -- Swing mechanism/RConn2 -- MSM and tooth plate3/RConn1
  Spatial force output1/RConn1 -- Flat tooth plate2/RConn1 -- Flat tooth plate/RConn1
  Flat tooth plate/LConn2 -- MSM and tooth plate1/LConn1 -- Swing mechanism/LConn1 -- Conn1/RConn1

== system MSM_strain_wave_actuator/MSM elements variant subsystem/Variable plate count Linear push push plates/Linear_swing_six_tooth_plates/Subsystem1 ==
  Control input [0; 1] : Inport
  Control input [0; 1]1 : Inport  Port=2
  Flat tooth plate : Flat_tooth_plate/Flat tooth plate  SystemSampleTime=-1  VariantActivationTime=update diagram  AllowFlexibleInterface=on  Latency=0  AutoFrameSizeCalculation=off
  Flat tooth plate2 : Flat_tooth_plate/Flat tooth plate  SystemSampleTime=-1  VariantActivationTime=update diagram  AllowFlexibleInterface=on  Latency=0  AutoFrameSizeCalculation=off
  MSM and tooth plate1 : MSM_element/MSM and tooth plate  PositionTargetValue=contraction_initial
  MSM and tooth plate3 : MSM_element/MSM and tooth plate  PositionTargetValue=contraction_initial
  Swing mechanism : Swing_mechanism/Swing mechanism  SystemSampleTime=-1  VariantActivationTime=update diagram  AllowFlexibleInterface=on  Latency=0  AutoFrameSizeCalculation=off
  Static frame 1 : PMIOPort  Side=Left
  Spatial force output1 : PMIOPort  Port=2  Side=Right
  Tooth Position Unit 1 : Outport
  "Tooth position COUNTERPHASE, mm" : Outport  Port=2
  wires:
  MSM and tooth plate1/1 -> Tooth Position Unit 1/1  "Tooth Position Unit 1"
  Control input [0; 1]1/1 -> MSM and tooth plate3/1
  MSM and tooth plate3/1 -> "Tooth position COUNTERPHASE, mm"/1
  Control input [0; 1]/1 -> MSM and tooth plate1/1
  connections:
  MSM and tooth plate1/LConn1 -- Static frame 1/RConn1 -- Flat tooth plate/LConn2 -- Swing mechanism/LConn1
  Flat tooth plate2/LConn2 -- MSM and tooth plate3/LConn1 -- Swing mechanism/LConn2
  MSM and tooth plate1/RConn1 -- Flat tooth plate/LConn1 -- Swing mechanism/RConn1
  Flat tooth plate2/LConn1 -- MSM and tooth plate3/RConn1 -- Swing mechanism/RConn2
  Spatial force output1/RConn1 -- Flat tooth plate2/RConn1 -- Flat tooth plate/RConn1

== system MSM_strain_wave_actuator/MSM elements variant subsystem/Variable plate count Linear push push plates/Linear_swing_six_tooth_plates/Subsystem2 ==
  Control input [0; 1] : Inport
  Control input [0; 1]1 : Inport  Port=2
  Flat tooth plate : Flat_tooth_plate/Flat tooth plate  SystemSampleTime=-1  VariantActivationTime=update diagram  AllowFlexibleInterface=on  Latency=0  AutoFrameSizeCalculation=off
  Flat tooth plate2 : Flat_tooth_plate/Flat tooth plate  SystemSampleTime=-1  VariantActivationTime=update diagram  AllowFlexibleInterface=on  Latency=0  AutoFrameSizeCalculation=off
  MSM and tooth plate1 : MSM_element/MSM and tooth plate  PositionTargetValue=contraction_initial
  MSM and tooth plate3 : MSM_element/MSM and tooth plate  PositionTargetValue=contraction_initial
  Swing mechanism : Swing_mechanism/Swing mechanism  SystemSampleTime=-1  VariantActivationTime=update diagram  AllowFlexibleInterface=on  Latency=0  AutoFrameSizeCalculation=off
  Static frame 1 : PMIOPort  Side=Left
  Spatial force output1 : PMIOPort  Port=2  Side=Right
  Tooth Position Unit 1 : Outport
  "Tooth position COUNTERPHASE, mm" : Outport  Port=2
  wires:
  MSM and tooth plate1/1 -> Tooth Position Unit 1/1  "Tooth Position Unit 1"
  Control input [0; 1]1/1 -> MSM and tooth plate3/1
  MSM and tooth plate3/1 -> "Tooth position COUNTERPHASE, mm"/1
  Control input [0; 1]/1 -> MSM and tooth plate1/1
  connections:
  MSM and tooth plate1/LConn1 -- Static frame 1/RConn1 -- Flat tooth plate/LConn2 -- Swing mechanism/LConn1
  Flat tooth plate2/LConn2 -- MSM and tooth plate3/LConn1 -- Swing mechanism/LConn2
  MSM and tooth plate1/RConn1 -- Flat tooth plate/LConn1 -- Swing mechanism/RConn1
  Flat tooth plate2/LConn1 -- MSM and tooth plate3/RConn1 -- Swing mechanism/RConn2
  Spatial force output1/RConn1 -- Flat tooth plate2/RConn1 -- Flat tooth plate/RConn1
